simulink model "r_hw_32"  (R2019a)
settings: Solver=VariableStepAuto  StartTime=0.0  StopTime=30  RelTol=1e-3
libraries: simulink x3
settings Model: Creator=Tamer  LastModifiedBy=Tamer

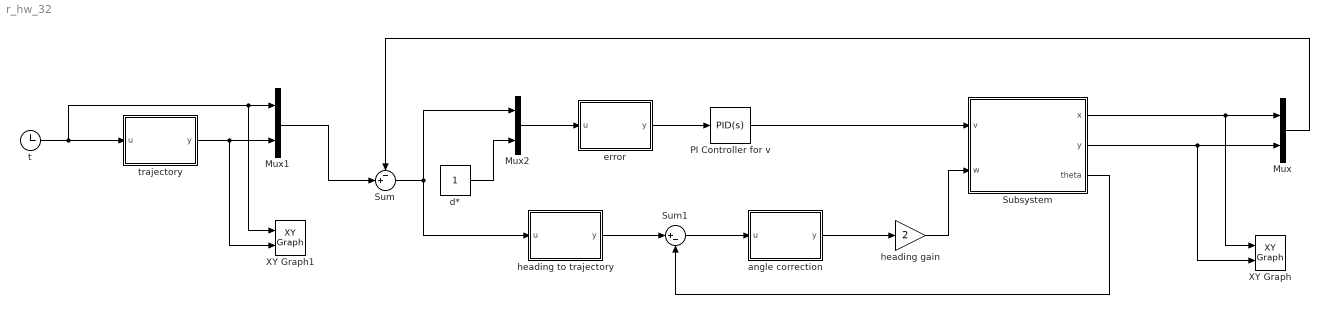
== system r_hw_32 ==
  Mux : Mux  Inputs=2
  Mux1 : Mux  Inputs=2
  Mux2 : Mux  Inputs=2
  PI Controller for v : simulink/Continuous/PID Controller  Controller=PID  Form=Parallel  TimeDomain=Continuous-time  SampleTime=-1  IntegratorMethod=Forward Euler  FilterMethod=Forward Euler  ControllerParametersSource=internal  P=0.5  I=0.1  D=0  UseFilter=on  N=100  TunerSelectOption=Transfer Function Based (PID Tuner App)  InitialConditionSource=internal  InitialConditionForIntegrator=0  InitialConditionForFilter=0  DifferentiatorICPrevScaledInput=0  ExternalReset=none  TrackingMode=off  Kt=1  LimitOutput=off  UpperSaturationLimit=inf  LowerSaturationLimit=-inf  LinearizeAsGain=on  AntiWindupMode=none  Kb=1  POutMin=[]  POutMax=[]  IOutMin=[]  IOutMax=[]  DOutMin=[]  DOutMax=[]  NOutMin=[]  NOutMax=[]  SumOutMin=[]  SumOutMax=[]  SaturationOutMin=[]  SaturationOutMax=[]  PParamMin=[]  PParamMax=[]  IParamMin=[]  IParamMax=[]  DParamMin=[]  DParamMax=[]  NParamMin=[]  NParamMax=[]  KbParamMin=[]  KbParamMax=[]  KtParamMin=[]  KtParamMax=[]  KbOutMin=[]  KbOutMax=[]  KtOutMin=[]  KtOutMax=[]  IntegratorOutMin=[]  IntegratorOutMax=[]  FilterOutMin=[]  FilterOutMax=[]  SumI1OutMin=[]  SumI1OutMax=[]  SumI2OutMin=[]  SumI2OutMax=[]  SumI3OutMin=[]  SumI3OutMax=[]  SumI4OutMin=[]  SumI4OutMax=[]  SumDOutMin=[]  SumDOutMax=[]  DifferentiatorOutMin=[]  DifferentiatorOutMax=[]  FilterDiffOutCoefMin=[]  FilterDiffOutCoefMax=[]  ReciprocalOutMin=[]  ReciprocalOutMax=[]  SumDenOutMin=[]  SumDenOutMax=[]  SumNumOutMin=[]  SumNumOutMax=[]  DivideOutMin=[]  DivideOutMax=[]  IntegratorContinuousStateAttributes=''  IntegratorStateMustResolveToSignalObject=off  IntegratorRTWStateStorageClass=Auto  FilterContinuousStateAttributes=''  FilterStateMustResolveToSignalObject=off  FilterRTWStateStorageClass=Auto  ParallelPVariant=InternalParameters  IdealPVariant=Disabled  IVariant=InternalParameters  DVariant=InternalParameters  IntegratorVariant=Continuous  SatVariant=Disabled  AWVariant=Passthrough  PCopyVariant=Disabled  TRVariant=Disabled  FdbkBlocksVariant=Forward  IdealPFdbkVariant=Disabled  SatFdbkVariant=Disabled  DerivativeFilterVariant=ContFilter  NVariant=InternalParameters  NCopyVariant=Disabled  FilterICVariant=InternalICsFilter  IntegratorICVariant=InternalICs  ExternalResetVariant=Disabled  TRSumVariant=Passthrough  SumFdbkVariant=Disabled  SumVariant=Sum_PID
  "Subsystem " : Subsystem
  Sum : Sum  Inputs=-+|
  Sum1 : Sum  Inputs=|+-
  XY Graph : simulink/Sinks/XY Graph  xmin=0  xmax=30  ymin=-2  ymax=2  st=-1
  XY Graph1 : simulink/Sinks/XY Graph  xmin=0  xmax=30  ymin=-2  ymax=2  st=-1
  angle correction : MATLAB Function  TreatAsAtomicUnit=on
  d* : Constant
  error : MATLAB Function  TreatAsAtomicUnit=on
  heading gain : Gain  Gain=2
  heading to trajectory : MATLAB Function  TreatAsAtomicUnit=on
  t : Clock
  trajectory : MATLAB Function  TreatAsAtomicUnit=on
  wires:
  Mux/1 -> Sum/1
  "Subsystem "/3(theta) -> Sum1/2
  Sum1/1 -> angle correction/1(u)
  heading to trajectory/1(y) -> Sum1/1
  angle correction/1(y) -> heading gain/1
  "Subsystem "/2(y) -> XY Graph/2, Mux/2
  heading gain/1 -> "Subsystem "/2(w)
  "Subsystem "/1(x) -> XY Graph/1, Mux/1
  error/1(y) -> PI Controller for v/1
  PI Controller for v/1 -> "Subsystem "/1(v)
  Mux1/1 -> Sum/2
  trajectory/1(y) -> XY Graph1/2, Mux1/2
  t/1 -> XY Graph1/1, Mux1/1, trajectory/1(u)
  Mux2/1 -> error/1(u)
  Sum/1 -> heading to trajectory/1(u), Mux2/1
  d*/1 -> Mux2/2

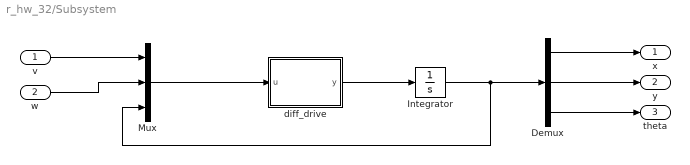
== system r_hw_32/Subsystem  ==
  v : Inport
  w : Inport  Port=2
  Demux : Demux  Outputs=3
  Integrator : Integrator  InitialCondition=[0;0;0]
  Mux : Mux  Inputs=3
  diff_drive : MATLAB Function  TreatAsAtomicUnit=on
  x : Outport
  y : Outport  Port=2
  theta : Outport  Port=3
  wires:
  v/1 -> Mux/1
  w/1 -> Mux/2
  Mux/1 -> diff_drive/1(u)
  diff_drive/1(y) -> Integrator/1
  Integrator/1 -> Mux/3, Demux/1
  Demux/1 -> x/1
  Demux/2 -> y/1
  Demux/3 -> theta/1

== matlab function r_hw_32/heading to trajectory ==
  data: u input; y output
function y = fcn(u)
%u(1) : x' - x
%u(2) : y' - y
y = atan2(u(2),u(1));

== matlab function r_hw_32/error ==
  data: u input; y output
function y = fcn(u)
%u(1) : x_traj - x
%u(2) : y_traj - y
%u(3) : d*
y = sqrt(u(1)^2+u(2)^2)-u(3);

== matlab function r_hw_32/angle correction ==
  data: u input; y output
function y = fcn(u)
%u(1) : theta* - theta
y = atan2(sin(u(1)),cos(u(1)));

== matlab function r_hw_32/Subsystem /diff_drive ==
  data: u input; y output
function y = fcn(u)
%u(1) : v
%u(2) : w
%u(3) : x
%u(4) : y
%u(5) : phi

y = [u(1)*cos(u(5)); u(1)*sin(u(5));u(2)];

== matlab function r_hw_32/trajectory ==
  data: u input; y output
function y = fcn(u)
%u(1) : t
y = cos(u(1));
